simulink model "Assignment3Question5"  (R2018a)
settings: Solver=FixedStepAuto  StartTime=0.0  StopTime=30  FixedStep=.01  RelTol=1e-3
settings Model: Creator=arjun  LastModifiedBy=arjun

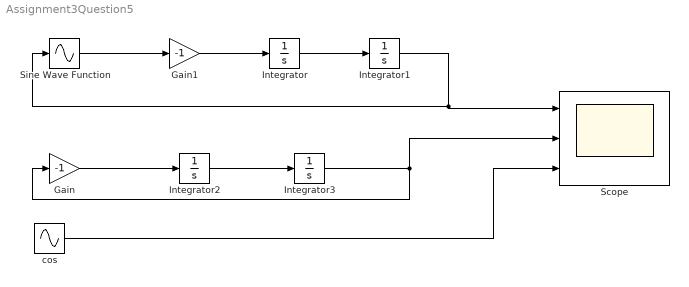
== system Assignment3Question5 ==
  Gain : Gain  Gain=-1
  Gain1 : Gain  Gain=-1
  Integrator : Integrator
  Integrator1 : Integrator  InitialCondition=1
  Integrator2 : Integrator
  Integrator3 : Integrator  InitialCondition=1
  Scope : Scope  NumInputPorts=3
  Sine Wave Function : Sin  TimeSource=Use external signal  SampleTime=0
  cos : Sin  Phase=pi/2  SampleTime=0
  wires:
  Sine Wave Function/1 -> Gain1/1
  Gain1/1 -> Integrator/1
  Integrator/1 -> Integrator1/1
  Integrator1/1 -> Scope/1, Sine Wave Function/1
  Gain/1 -> Integrator2/1
  Integrator2/1 -> Integrator3/1
  Integrator3/1 -> Scope/2, Gain/1
  cos/1 -> Scope/3
